simulink model "momentumBasedFlight"  (R2021b)
settings: Solver=VariableStepAuto  StartTime=0.0  StopTime=Config.simulationTime  RelTol=1e-3
InitFcn:
  | cd(fileparts(which(bdroot)));
  | initMomentumBasedFlight;
StopFcn:
  | cd(fileparts(which(bdroot)));
  | stopMomentumBasedFlight;
undefined symbols (not defined in the file or in its folder): aero_config, biasVectorConstraint_feet, Config, ConstraintMatrix_feet, DiscIntNeverNeededParam, frameNames, Frames
libraries: WBToolboxLibrary x104, momentum_flight_control_sublib x4, thrust_estimation_sublib x1, jets_control x1
(part 1 of 3)
settings Model: NumberOfSteps=50  Creator=apaolino  LastModifiedBy=icub
settings SolverCC: AlgebraicLoopSolver=TrustRegion
settings OptimizationCC: BlockReduction=off  BooleanDataType=off
settings DebuggingCC: SaveWithParameterizedLinksMsg=none  UnderspecifiedInitializationDetection=Classic  MergeDetectMultiDrivingBlocksExec=none  SignalResolutionControl=TryResolveAllWithWarning  UnconnectedInputMsg=none  UnconnectedOutputMsg=none  UnconnectedLineMsg=none
settings HardwareCC: TargetUnknown=on
settings ModelReferenceCC: EnableRefExpFcnMdlSchedulingChecks=off  PropagateSignalLabelsOutOfModel=off

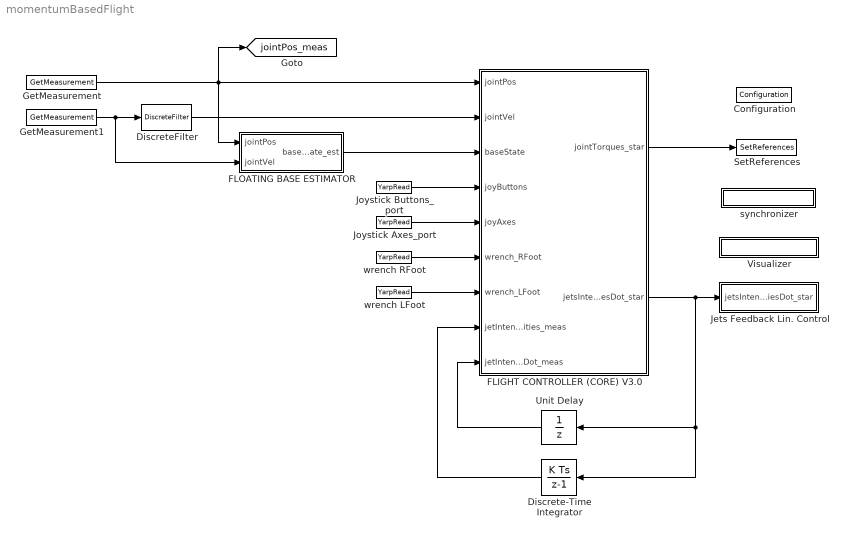
== system momentumBasedFlight ==
  Configuration : WBToolboxLibrary/Utilities/Configuration  ConfigSource=Workspace  ConfigObject='WBTConfigRobot'
      settings: SourceProductName=WholeBodyToolbox
  Discrete-Time Integrator : DiscreteIntegrator  InitialCondition=Config.initialConditions.jets_thrust  SampleTime=-1  ICPrevOutput=DiscIntNeverNeededParam  ICPrevScaledInput=DiscIntNeverNeededParam
  DiscreteFilter : WBToolboxLibrary/Utilities/DiscreteFilter  filterType=FirstOrderLowPassFilter  numCoeffs=[0]  denCoeffs=[0]  Fc=3  Ts=Config.tStep  orderMedianFilter=0  initStatus=on  y0=zeros(23,1)  u0=[0]
      settings: SourceProductName=WholeBodyToolbox
  FLIGHT CONTROLLER (CORE) V3.0 : Subsystem
  FLOATING BASE ESTIMATOR : Subsystem
  GetMeasurement : WBToolboxLibrary/States/GetMeasurement  measuredType=Joints Position
      settings: SourceProductName=WholeBodyToolbox
  GetMeasurement1 : WBToolboxLibrary/States/GetMeasurement  measuredType=Joints Velocity
      settings: SourceProductName=WholeBodyToolbox
  Jets Feedback Lin. Control : Subsystem
  Joystick Axes_port : WBToolboxLibrary/Utilities/YarpRead  portName=Ports.JOYSTICK_AXIS  signalSize=6  timeout=0.5  blocking=off  timestamp=off  autoconnect=on  errorOnConnection=off
      settings: SourceProductName=WholeBodyToolbox
  Joystick Buttons_port : WBToolboxLibrary/Utilities/YarpRead  portName=Ports.JOYSTICK_BUTTONS  signalSize=24  timeout=0.5  blocking=off  timestamp=off  autoconnect=on  errorOnConnection=off
      settings: SourceProductName=WholeBodyToolbox
  SetReferences : WBToolboxLibrary/Actuators/SetReferences  controlType=Torque  refSpeed=10*(pi/180)  refAcceleration=1000000*(pi/180)
      settings: SourceProductName=WholeBodyToolbox
  Unit Delay : UnitDelay  SampleTime=-1  HasFrameUpgradeWarning=on
  Visualizer : Subsystem
      mask Display: disp('VISUALIZER')
  synchronizer : Subsystem
      mask Display: disp('SYNCHRONIZER')
  wrench LFoot : WBToolboxLibrary/Utilities/YarpRead  portName=Ports.WRENCH_LEFT_FOOT  signalSize=6  timeout=0.5  blocking=off  timestamp=off  autoconnect=on  errorOnConnection=on
      settings: SourceProductName=WholeBodyToolbox
  wrench RFoot : WBToolboxLibrary/Utilities/YarpRead  portName=Ports.WRENCH_RIGHT_FOOT  signalSize=6  timeout=0.5  blocking=off  timestamp=off  autoconnect=on  errorOnConnection=on
      settings: SourceProductName=WholeBodyToolbox
  tag scope: jointPos_meas=global
  wires:
  GetMeasurement/1 -> FLIGHT CONTROLLER (CORE) V3.0/1(jointPos), [jointPos_meas], FLOATING BASE ESTIMATOR/1(jointPos)
  GetMeasurement1/1 -> DiscreteFilter/1, FLOATING BASE ESTIMATOR/2(jointVel)
  Joystick Buttons_port/1 -> FLIGHT CONTROLLER (CORE) V3.0/4(joyButtons)
  Joystick Axes_port/1 -> FLIGHT CONTROLLER (CORE) V3.0/5(joyAxes)
  wrench LFoot/1 -> FLIGHT CONTROLLER (CORE) V3.0/7(wrench_LFoot)
  wrench RFoot/1 -> FLIGHT CONTROLLER (CORE) V3.0/6(wrench_RFoot)
  FLIGHT CONTROLLER (CORE) V3.0/1(jointTorques_star) -> SetReferences/1
  FLIGHT CONTROLLER (CORE) V3.0/2(jetsIntensitiesDot_star) -> Jets Feedback Lin. Control/1(jetsIntensitiesDot_star), Discrete-Time Integrator/1, Unit Delay/1
  Unit Delay/1 -> FLIGHT CONTROLLER (CORE) V3.0/9(jetIntensitiesDot_meas)
  Discrete-Time Integrator/1 -> FLIGHT CONTROLLER (CORE) V3.0/8(jetIntensities_meas)
  FLOATING BASE ESTIMATOR/1(baseState_est) -> FLIGHT CONTROLLER (CORE) V3.0/3(baseState)
  DiscreteFilter/1 -> FLIGHT CONTROLLER (CORE) V3.0/2(jointVel)

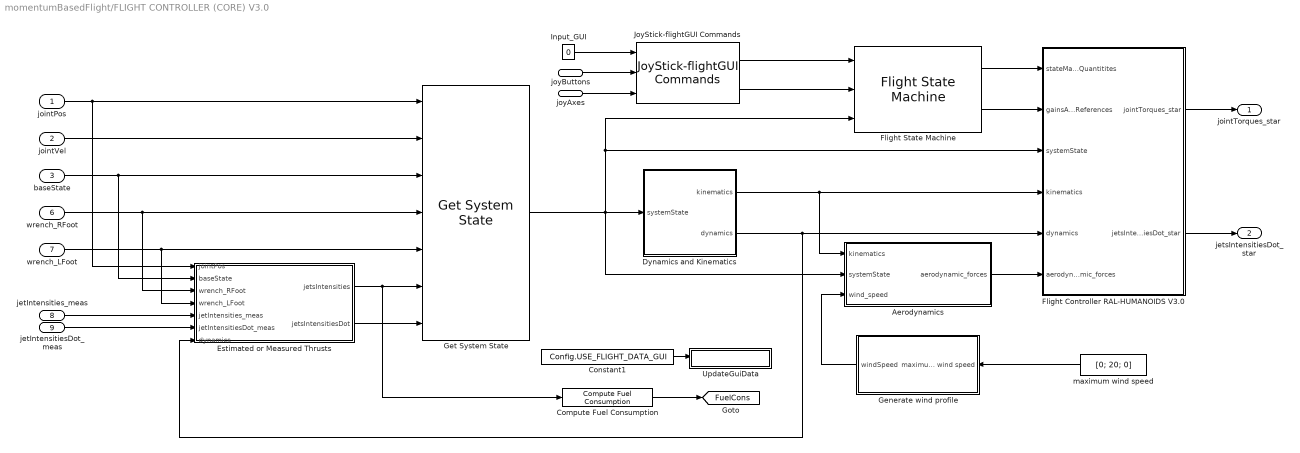
== system momentumBasedFlight/FLIGHT CONTROLLER (CORE) V3.0 ==
  jointPos : Inport
  jointVel : Inport  Port=2
  baseState : Inport  Port=3
  joyButtons : Inport  Port=4
  joyAxes : Inport  Port=5
  wrench_RFoot : Inport  Port=6
  wrench_LFoot : Inport  Port=7
  jetIntensities_meas : Inport  Port=8
  jetIntensitiesDot_meas : Inport  Port=9
  Aerodynamics : Subsystem
  Compute Fuel Consumption : momentum_flight_control_sublib/Compute Fuel Consumption  Parameter1=Config
      settings: SourceProductName=iRonCub Library
  Constant1 : Constant  Value=Config.USE_FLIGHT_DATA_GUI
  Dynamics and Kinematics : Subsystem  AncestorBlock=momentum_flight_control_sublib/Dynamics and Kinematics  mask{Parameter1=Config, Parameter2=Frames}
      mask prompts: Parameter1 "Specify the parameters struct"; Parameter2 "Specify the frame names struct"
      mask DialogControl DescGroupVar Prompt: Dynamics and Kinematics
      mask DialogControl DescTextVar Prompt: Computes the dynamics and kinematics quantities that are required by the iRonCub flight controller.
  Estimated or Measured Thrusts : Subsystem
  Flight Controller RAL-HUMANOIDS V3.0 : Subsystem  mask{Parameter1=Config}
      mask prompts: Parameter1 "Specify the parameters struct"
      mask DialogControl DescGroupVar Prompt: Flight Controller RAL-HUMANOIDS
      mask DialogControl DescTextVar Prompt: This block implements the momentum-based flight controller decribed in RAL 2018 and HUMANOIDS 2018 papers.
      mask DialogControl Control3 Prompt: References:
      mask DialogControl Control5 Prompt: RAL 2018 paper
      mask DialogControl Control5 Callback: web https://ieeexplore.ieee.org/document/7997895
      mask DialogControl Control6 Prompt: HUMANOIDS 2018 paper
      mask DialogControl Control6 Callback: web https://ieeexplore.ieee.org/document/8624985
  Flight State Machine : momentum_flight_control_sublib/Flight State Machine  Parameter1=Config  Parameter2=Frames
      settings: SourceProductName=iRonCub Library
  Generate wind profile : Subsystem
  Get System State : momentum_flight_control_sublib/Get System State  Parameter1=Frames
      settings: SourceProductName=iRonCub Library
  Input_GUI : Constant  Value=0
  JoyStick-flightGUI Commands : momentum_flight_control_sublib/JoyStick-flightGUI Commands  Parameter1=Config
      link override Input_GUI: Value=0
      settings: SourceProductName=iRonCub Library
  UpdateGuiData : Subsystem
      mask Display: disp('Update Data GUI')
  maximum wind speed : Constant  Value=[0; 20; 0]
  jointTorques_star : Outport  VectorParamsAs1DForOutWhenUnconnected=off
  jetsIntensitiesDot_star : Outport  Port=2  VectorParamsAs1DForOutWhenUnconnected=off
  tag scope: FuelCons=global
  wires:
  wrench_LFoot/1 -> Get System State/5, Estimated or Measured Thrusts/4(wrench_LFoot)
  Flight Controller RAL-HUMANOIDS V3.0/2(jetsIntensitiesDot_star) -> jetsIntensitiesDot_star/1
  Flight Controller RAL-HUMANOIDS V3.0/1(jointTorques_star) -> jointTorques_star/1
  Get System State/1 -> Dynamics and Kinematics/1(systemState), Aerodynamics/2(systemState), Flight Controller RAL-HUMANOIDS V3.0/3(systemState), Flight State Machine/3
  jointVel/1 -> Get System State/2
  jointPos/1 -> Get System State/1, Estimated or Measured Thrusts/1(jointPos)
  wrench_RFoot/1 -> Get System State/4, Estimated or Measured Thrusts/3(wrench_RFoot)
  baseState/1 -> Get System State/3, Estimated or Measured Thrusts/2(baseState)
  Compute Fuel Consumption/1 -> [FuelCons]
  JoyStick-flightGUI Commands/1 -> Flight State Machine/1
  JoyStick-flightGUI Commands/2 -> Flight State Machine/2
  Flight State Machine/1 -> Flight Controller RAL-HUMANOIDS V3.0/1(stateMachineQuantitites)
  Flight State Machine/2 -> Flight Controller RAL-HUMANOIDS V3.0/2(gainsAndReferences)
  joyAxes/1 -> JoyStick-flightGUI Commands/3
  joyButtons/1 -> JoyStick-flightGUI Commands/2
  Input_GUI/1 -> JoyStick-flightGUI Commands/1
  Constant1/1 -> UpdateGuiData/Enable
  jetIntensities_meas/1 -> Estimated or Measured Thrusts/5(jetIntensities_meas)
  jetIntensitiesDot_meas/1 -> Estimated or Measured Thrusts/6(jetIntensitiesDot_meas)
  Estimated or Measured Thrusts/1(jetsIntensities) -> Compute Fuel Consumption/1, Get System State/6
  Estimated or Measured Thrusts/2(jetsIntensitiesDot) -> Get System State/7
  Generate wind profile/1(windSpeed) -> Aerodynamics/3(wind_speed)
  maximum wind speed/1 -> Generate wind profile/1(maximum wind speed)
  Dynamics and Kinematics/2(dynamics) -> Estimated or Measured Thrusts/7(dynamics), Flight Controller RAL-HUMANOIDS V3.0/5(dynamics)
  Dynamics and Kinematics/1(kinematics) -> Flight Controller RAL-HUMANOIDS V3.0/4(kinematics), Aerodynamics/1(kinematics)
  Aerodynamics/1(aerodynamic_forces) -> Flight Controller RAL-HUMANOIDS V3.0/6(aerodynamic_forces)

== system momentumBasedFlight/FLOATING BASE ESTIMATOR ==
  jointPos : Inport
  jointVel : Inport  Port=2
  Compute State Velocity : Subsystem
  Compute base to fixed link transform : Subsystem
  Constant : Constant  Value=[1, 1]
  IMU_meas : WBToolboxLibrary/Utilities/YarpRead  portName=Ports.IMU  signalSize=Ports.IMU_PORT_SIZE  timeout=0.5  blocking=off  timestamp=off  autoconnect=on  errorOnConnection=off
      settings: SourceProductName=WholeBodyToolbox
  Terminator : Terminator
  baseState_feetFixed : MATLAB Function  TreatAsAtomicUnit=on
  baseState_est : Outport
  wires:
  IMU_meas/1 -> Compute base to fixed link transform/2(IMU_meas)
  jointPos/1 -> Compute State Velocity/1(jointPos), Compute base to fixed link transform/1(jointPos)
  jointVel/1 -> Compute State Velocity/2(jointVel)
  Constant/1 -> Compute State Velocity/4("feetContactStatus ")
  Compute base to fixed link transform/1(fixed_l_sole_H_b) -> baseState_feetFixed/2(w_H_b_yoga), Compute State Velocity/3(w_H_b)
  Compute base to fixed link transform/2(fixed_r_sole_H_b) -> Terminator/1
  Compute State Velocity/1(nu) -> baseState_feetFixed/1(nu)
  baseState_feetFixed/1(outBaseState) -> baseState_est/1

== system momentumBasedFlight/Jets Feedback Lin. Control ==
  jetsIntensitiesDot_star : Inport
  Bus Creator : BusCreator  Inputs=2
  Feedback Linearization Jets Control : jets_control/Feedback linearization 4-jets control  Conf=Config
      settings: SourceProductName=iRonCub Library
  Logical Operator : Logic  Operator=NOT  AllPortsSameDT=off  OutDataTypeStr=boolean
  "ON_GAZEBO " : Constant  Value=Config.USE_JET_DYNAMICS
  SET THROTTLE : Subsystem  Commented=on
  SET_THRUST_DERIVATIVE : Subsystem  Commented=on
  tag scope: throttle=global
  wires:
  jetsIntensitiesDot_star/1 -> Feedback Linearization Jets Control/2, SET_THRUST_DERIVATIVE/1(jetsIntensitiesDot_star)
  Feedback Linearization Jets Control/1 -> [throttle], SET THROTTLE/1(throttle)
  Bus Creator/1 -> Feedback Linearization Jets Control/1
  [jetsIntensities] -> Bus Creator/1  "jetIntensitiesFiltered"
  [jetIntensitiesDot] -> Bus Creator/2  "jetDerivativesEst"
  "ON_GAZEBO "/1 -> SET THROTTLE/Enable, Logical Operator/1
  Logical Operator/1 -> SET_THRUST_DERIVATIVE/Enable

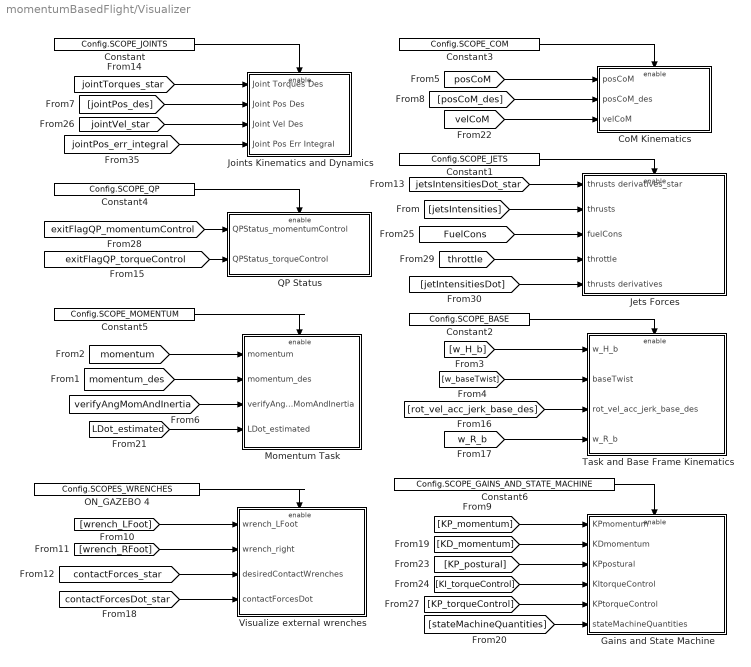
== system momentumBasedFlight/Visualizer ==
  CoM Kinematics : Subsystem
  Constant : Constant  Value=Config.SCOPE_JOINTS
  Constant1 : Constant  Value=Config.SCOPE_JETS
  Constant2 : Constant  Value=Config.SCOPE_BASE
  Constant3 : Constant  Value=Config.SCOPE_COM
  Constant4 : Constant  Value=Config.SCOPE_QP
  Constant5 : Constant  Value=Config.SCOPE_MOMENTUM
  Constant6 : Constant  Value=Config.SCOPE_GAINS_AND_STATE_MACHINE
  Gains and State Machine : Subsystem
  Jets Forces : Subsystem
  Joints Kinematics and Dynamics : Subsystem
  Momentum Task : Subsystem
  ON_GAZEBO 4 : Constant  Value=Config.SCOPES_WRENCHES
  QP Status : Subsystem
  Task and Base Frame Kinematics : Subsystem
  "Visualize external wrenches  " : Subsystem
  wires:
  [jointTorques_star] -> Joints Kinematics and Dynamics/1(Joint Torques Des)
  [jointPos_des] -> Joints Kinematics and Dynamics/2(Joint Pos Des)
  [w_H_b] -> Task and Base Frame Kinematics/1(w_H_b)
  [jointVel_star] -> Joints Kinematics and Dynamics/3(Joint Vel Des)
  Constant/1 -> Joints Kinematics and Dynamics/Enable
  [jetsIntensitiesDot_star] -> Jets Forces/1(thrusts derivatives_star)
  Constant1/1 -> Jets Forces/Enable
  [w_baseTwist] -> Task and Base Frame Kinematics/2(baseTwist)
  Constant2/1 -> Task and Base Frame Kinematics/Enable
  [momentum] -> Momentum Task/1(momentum)
  [posCoM] -> CoM Kinematics/1(posCoM)
  [posCoM_des] -> CoM Kinematics/2(posCoM_des)
  Constant3/1 -> CoM Kinematics/Enable
  [exitFlagQP_momentumControl] -> QP Status/1(QPStatus_momentumControl)
  Constant4/1 -> QP Status/Enable
  Constant5/1 -> Momentum Task/Enable
  [rot_vel_acc_jerk_base_des] -> Task and Base Frame Kinematics/3(rot_vel_acc_jerk_base_des)
  [w_R_b] -> Task and Base Frame Kinematics/4(w_R_b)
  [momentum_des] -> Momentum Task/2(momentum_des)
  [jetsIntensities] -> Jets Forces/2(thrusts)
  [verifyAngMomAndInertia] -> Momentum Task/3(verifyAngMomAndInertia)
  [wrench_LFoot] -> "Visualize external wrenches  "/1(wrench_LFoot)
  [wrench_RFoot] -> "Visualize external wrenches  "/2(wrench_right)
  ON_GAZEBO 4/1 -> "Visualize external wrenches  "/Enable
  [contactForces_star] -> "Visualize external wrenches  "/3(desiredContactWrenches)
  [exitFlagQP_torqueControl] -> QP Status/2(QPStatus_torqueControl)
  [contactForcesDot_star] -> "Visualize external wrenches  "/4(contactForcesDot)
  [LDot_estimated] -> Momentum Task/4(LDot_estimated)
  Constant6/1 -> Gains and State Machine/Enable
  [KP_momentum] -> Gains and State Machine/1(KPmomentum)
  [stateMachineQuantities] -> Gains and State Machine/6(stateMachineQuantities)
  [KD_momentum] -> Gains and State Machine/2(KDmomentum)
  [KP_postural] -> Gains and State Machine/3(KPpostural)
  [KP_torqueControl] -> Gains and State Machine/5(KPtorqueControl)
  [KI_torqueControl] -> Gains and State Machine/4(KItorqueControl)
  [jointPos_err_integral] -> Joints Kinematics and Dynamics/4(Joint Pos Err Integral)
  [velCoM] -> CoM Kinematics/3(velCoM)
  [FuelCons] -> Jets Forces/3(fuelCons)
  [throttle] -> Jets Forces/4(throttle)
  [jetIntensitiesDot] -> Jets Forces/5(thrusts derivatives)

== system momentumBasedFlight/synchronizer ==
  GAZEBO_SYNCHRONIZER : Subsystem
  Logical Operator : Logic  Operator=NOT  AllPortsSameDT=off  OutDataTypeStr=boolean
  "ON_GAZEBO " : Constant  Value=Config.ON_GAZEBO
  REAL_TIME_SYNC : Subsystem
  wires:
  Logical Operator/1 -> REAL_TIME_SYNC/Enable
  "ON_GAZEBO "/1 -> GAZEBO_SYNCHRONIZER/Enable, Logical Operator/1

== system momentumBasedFlight/FLIGHT CONTROLLER (CORE) V3.0/Aerodynamics ==
  kinematics : Inport
  systemState : Inport  Port=2
  wind_speed : Inport  Port=3
  Bus Selector : BusSelector  OutputSignals=w_baseTwist,jointVel
  Bus Selector1 : BusSelector  OutputSignals=J_aeroForce,matrixOfLinkCoMTransform
  Terminator : Terminator
  aeroDyn : MATLABSystem  System=aeroDyn  aero_config=aero_config_with_frames  SimulateUsing=Interpreted execution
      mask Type: aeroDyn
      mask Display:
      | disp('aeroDyn');
      | port_label('input',1,'base_velocity');
      | port_label('input',2,'joints_velocity');
      | port_label('input',3,'wind_speed');
      | port_label('input',4,'J_aeroForce');
      | port_label('input',5,'matrixOfAeroTransform');
      | port_label('output',1,'aerodynamic_forces');
      | port_label('output',2,'generalized_aerodynamic_wrench');
  aerodynamic_forces : Outport
  wires:
  systemState/1 -> Bus Selector/1
  Bus Selector/1 -> aeroDyn/1  "<w_baseTwist>"
  aeroDyn/1 -> aerodynamic_forces/1  "aerodynamic_forces"
  aeroDyn/2 -> Terminator/1
  kinematics/1 -> Bus Selector1/1
  Bus Selector1/1 -> aeroDyn/4  "<J_aeroForce>"
  Bus Selector1/2 -> aeroDyn/5  "<matrixOfLinkCoMTransform>"
  Bus Selector/2 -> aeroDyn/2  "<jointVel>"
  wind_speed/1 -> aeroDyn/3

== system momentumBasedFlight/FLIGHT CONTROLLER (CORE) V3.0/Dynamics and Kinematics ==
  systemState : Inport
  Bus Creator1 : BusCreator  Inputs=5
  Bus Creator2 : BusCreator  Inputs=15
  Bus Selector : BusSelector  OutputSignals=w_H_b,jointPos,w_baseTwist,jointVel
  Dynamic Quantities : Subsystem
  Kinematic Quantities : Subsystem
  kinematics : Outport  VectorParamsAs1DForOutWhenUnconnected=off
  dynamics : Outport  Port=2  VectorParamsAs1DForOutWhenUnconnected=off
  wires:
  Dynamic Quantities/5(w_I_c) -> Bus Creator1/5  "w_I_c"
  Kinematic Quantities/12(posCoM) -> Dynamic Quantities/1(posCoM), Bus Creator2/12  "posCoM"
  Kinematic Quantities/11(matrixOfJetsArms) -> Bus Creator2/11  "matrixOfJetsArms"
  Kinematic Quantities/10(matrixOfJetsAxes) -> Bus Creator2/10  "matrixOfJetAxes"
  Kinematic Quantities/9(w_H_RFoot) -> Bus Creator2/9  "w_H_RFoot"
  Kinematic Quantities/8(w_H_LFoot) -> Bus Creator2/8  "w_H_LFoot"
  Kinematic Quantities/7(JDot_RFoot_nu) -> Bus Creator2/7  "JDot_RFoot_nu"
  Kinematic Quantities/6(JDot_LFoot_nu) -> Bus Creator2/6  "JDot_LFoot_nu"
  Kinematic Quantities/5(J_RFoot) -> Bus Creator2/5  "J_RFoot"
  Kinematic Quantities/4(J_LFoot) -> Bus Creator2/4  "J_LFoot"
  Kinematic Quantities/3(w_R_b) -> Bus Creator2/3  "w_R_b"
  Kinematic Quantities/2(J_CoM) -> Bus Creator2/2  "J_CoM"
  Kinematic Quantities/1(J_jets) -> Bus Creator2/1  "J_jets"
  Bus Creator2/1 -> kinematics/1
  Bus Creator1/1 -> dynamics/1
  Dynamic Quantities/1(M) -> Bus Creator1/1  "M"
  Dynamic Quantities/2("h ") -> Bus Creator1/2  "h"
  Dynamic Quantities/3(L) -> Bus Creator1/3  "L"
  Dynamic Quantities/4(CMM) -> Bus Creator1/4  "CMM"
  Bus Selector/4 -> Kinematic Quantities/4(jointVel), Dynamic Quantities/5(jointVel)  "<jointVel>"
  Bus Selector/3 -> Kinematic Quantities/3(w_baseTwist), Dynamic Quantities/4(w_baseTwist)  "<w_baseTwist>"
  Bus Selector/2 -> Kinematic Quantities/2(jointPos), Dynamic Quantities/3(jointPos)  "<jointPos>"
  Bus Selector/1 -> Kinematic Quantities/1(w_H_b), Dynamic Quantities/2(w_H_b)  "<w_H_b>"
  systemState/1 -> Bus Selector/1
  Kinematic Quantities/13(matrixOfAeroArms) -> Bus Creator2/13
  Kinematic Quantities/14(J_aeroForces) -> Bus Creator2/14  "J_aeroForce"
  Kinematic Quantities/15(matrixOfAeroTransform) -> Bus Creator2/15

== system momentumBasedFlight/FLIGHT CONTROLLER (CORE) V3.0/Estimated or Measured Thrusts ==
  jointPos : Inport
  baseState : Inport  Port=2
  wrench_RFoot : Inport  Port=3
  wrench_LFoot : Inport  Port=4
  jetIntensities_meas : Inport  Port=5
  jetIntensitiesDot_meas : Inport  Port=6
  dynamics : Inport  Port=7
  " Thrust Estimator" : Subsystem
  "ON_GAZEBO " : Constant  Value=Config.USE_JET_DYNAMICS
  ON_GAZEBO 1 : Constant  Value=Config.USE_THRUST_ESTIMATOR
  Selector1 : Selector  InputPortWidth=18  IndexOptions=Index vector (dialog)  Indices=[1:6]  OutputSizes=1
  Switch : Switch  Criteria=u2 > Threshold
  Switch1 : Switch  Criteria=u2 > Threshold
  fromPosRPYtoTransfMatrix : MATLAB Function  TreatAsAtomicUnit=on
  jetsIntensities : Outport
  jetsIntensitiesDot : Outport  Port=2
  wires:
  Switch/1 -> jetsIntensities/1  "jetsIntensities"
  jetIntensitiesDot_meas/1 -> Switch1/3
  " Thrust Estimator"/1(jetIntensities_Estimated) -> Switch/1
  jetIntensities_meas/1 -> Switch/3
  " Thrust Estimator"/2(jetIntensitiesDot_Estimated) -> Switch1/1
  wrench_RFoot/1 -> " Thrust Estimator"/5(wrench_RFoot)
  ON_GAZEBO 1/1 -> Switch/2, Switch1/2
  jointPos/1 -> " Thrust Estimator"/2(jointPos)
  Switch1/1 -> jetsIntensitiesDot/1  "jetsIntensitiesDot"
  dynamics/1 -> " Thrust Estimator"/3(dynamics)
  [throttle] -> " Thrust Estimator"/6(throttle)
  "ON_GAZEBO "/1 -> " Thrust Estimator"/Enable
  wrench_LFoot/1 -> " Thrust Estimator"/4(wrench_LFoot)
  baseState/1 -> Selector1/1
  fromPosRPYtoTransfMatrix/1(w_H_b) -> " Thrust Estimator"/1(w_H_b)
  Selector1/1 -> fromPosRPYtoTransfMatrix/1(pos_rpy)

== system momentumBasedFlight/FLIGHT CONTROLLER (CORE) V3.0/Flight Controller RAL-HUMANOIDS V3.0 ==
  stateMachineQuantitites : Inport
  gainsAndReferences : Inport  Port=2
  systemState : Inport  Port=3
  kinematics : Inport  Port=4
  dynamics : Inport  Port=5
  aerodynamic_forces : Inport  Port=6
  Discrete-Time Integrator : DiscreteIntegrator  Commented=on  InitialConditionSource=external  SampleTime=Config.tStep  ICPrevOutput=DiscIntNeverNeededParam  ICPrevScaledInput=DiscIntNeverNeededParam
  GetMeasurement : WBToolboxLibrary/States/GetMeasurement  Commented=on  measuredType=Joints Position
      settings: SourceProductName=WholeBodyToolbox
  Joint Torque Control for Flying : Subsystem
  Momentum Control for Flying : Subsystem
  SetReferences : WBToolboxLibrary/Actuators/SetReferences  Commented=on  controlType=Position Direct  refSpeed=10*(pi/180)  refAcceleration=1000000*(pi/180)
      settings: SourceProductName=WholeBodyToolbox
  deadZone : Subsystem  Commented=on
  "holder " : WBToolboxLibrary/Utilities/holder   Commented=on
      settings: SourceProductName=WholeBodyToolbox
  jointTorques_star : Outport  VectorParamsAs1DForOutWhenUnconnected=off
  jetsIntensitiesDot_star : Outport  Port=2  VectorParamsAs1DForOutWhenUnconnected=off
  tag scope: jointTorques_star=global
  wires:
  Momentum Control for Flying/3(jetsIntensitiesDot_star) -> jetsIntensitiesDot_star/1
  Joint Torque Control for Flying/1(jointTorques_star) -> [jointTorques_star], jointTorques_star/1
  Momentum Control for Flying/2(contactForces_star) -> Joint Torque Control for Flying/2(contactForces_star)
  dynamics/1 -> Momentum Control for Flying/5(dynamics), Joint Torque Control for Flying/7(dynamics)
  kinematics/1 -> Momentum Control for Flying/4(kinematics), Joint Torque Control for Flying/6(kinematics)
  systemState/1 -> Momentum Control for Flying/3(systemState), Joint Torque Control for Flying/5(systemState)
  gainsAndReferences/1 -> Joint Torque Control for Flying/4(gainsAndReferences), Momentum Control for Flying/2(gainsAndReferences)
  stateMachineQuantitites/1 -> Joint Torque Control for Flying/3(stateMachineQuantitites), Momentum Control for Flying/1(stateMachineQuantitites)
  aerodynamic_forces/1 -> Joint Torque Control for Flying/8(aerodynamic_forces), Momentum Control for Flying/6(aerodynamic_forces)
  "holder "/1 -> Discrete-Time Integrator/2
  Discrete-Time Integrator/1 -> SetReferences/1
  GetMeasurement/1 -> "holder "/1
  deadZone/1(u_cut) -> Discrete-Time Integrator/1
  Momentum Control for Flying/1(jointVel_star) -> Joint Torque Control for Flying/1(jointVel_star), deadZone/1(u)

== system momentumBasedFlight/FLIGHT CONTROLLER (CORE) V3.0/Generate wind profile ==
  maximum wind speed : Inport
  Clock : Clock
  Constant1 : Constant  Value=aero_config.USE_WIND_SPEED
  MATLAB Function : MATLAB Function  TreatAsAtomicUnit=on
  Switch1 : Switch  Criteria=u2 ~= 0
  wind speed : Scope
  zero_wind_speed : Constant  Value=zeros(3,1)
  windSpeed : Outport
  tag scope: windSpeed=global
  wires:
  Clock/1 -> MATLAB Function/2(time)
  zero_wind_speed/1 -> Switch1/3
  maximum wind speed/1 -> MATLAB Function/1(maxWindSpeed)
  MATLAB Function/1(windSpeed) -> wind speed/1, [windSpeed], Switch1/1
  Constant1/1 -> Switch1/2
  Switch1/1 -> windSpeed/1

== system momentumBasedFlight/FLIGHT CONTROLLER (CORE) V3.0/UpdateGuiData ==
  Enable : EnablePort
  Clock : Clock
  Update Data for the GUI : MATLAB Function  TreatAsAtomicUnit=on
  wires:
  Clock/1 -> Update Data for the GUI/1(time)

== system momentumBasedFlight/FLOATING BASE ESTIMATOR/Compute State Velocity ==
  jointPos : Inport
  jointVel : Inport  Port=2
  w_H_b : Inport  Port=3
  "feetContactStatus " : Inport  Port=4
  Compute Base Velocity : MATLAB Function  TreatAsAtomicUnit=on
  Feet Jacobians : Subsystem
  Mux : Mux  Inputs=2
  nu : Outport  VectorParamsAs1DForOutWhenUnconnected=off
  wires:
  jointVel/1 -> Mux/2, Compute Base Velocity/4(jointVel)
  Mux/1 -> nu/1
  "feetContactStatus "/1 -> Compute Base Velocity/3(feetContactStatus)
  Compute Base Velocity/1(nu_b) -> Mux/1
  jointPos/1 -> Feet Jacobians/1(jointPos)
  w_H_b/1 -> Feet Jacobians/2(w_H_b)
  Feet Jacobians/1(J_l_sole) -> Compute Base Velocity/1(J_l_sole)
  Feet Jacobians/2(J_r_sole) -> Compute Base Velocity/2(J_r_sole)

== system momentumBasedFlight/FLOATING BASE ESTIMATOR/Compute base to fixed link transform ==
  jointPos : Inport
  IMU_meas : Inport  Port=2
  Constant7 : Constant  Value=eye(4)
  "LFoot to base link transform " : Subsystem
  RFoot to base link transform : Subsystem
  Relative transform l_sole_H_base : WBToolboxLibrary/Model/Kinematics/ForwardKinematics  frameName=Frames.LFOOT_FRAME
      settings: SourceProductName=WholeBodyToolbox
  Relative transform r_sole_H_base : WBToolboxLibrary/Model/Kinematics/ForwardKinematics  frameName=Frames.RFOOT_FRAME
      settings: SourceProductName=WholeBodyToolbox
  fixed_l_sole_H_b : Outport  VectorParamsAs1DForOutWhenUnconnected=off
  fixed_r_sole_H_b : Outport  Port=2  VectorParamsAs1DForOutWhenUnconnected=off
  wires:
  Constant7/1 -> RFoot to base link transform/4(w_H_base_fixed), "LFoot to base link transform "/4(w_H_base_fixed), Relative transform r_sole_H_base/1, Relative transform l_sole_H_base/1
  RFoot to base link transform/1(link_H_b) -> fixed_r_sole_H_b/1
  "LFoot to base link transform "/1(link_H_b) -> fixed_l_sole_H_b/1
  Relative transform l_sole_H_base/1 -> "LFoot to base link transform "/3(w_H_link)
  Relative transform r_sole_H_base/1 -> RFoot to base link transform/3(w_H_link)
  jointPos/1 -> RFoot to base link transform/1(jointPos), "LFoot to base link transform "/1(jointPos), Relative transform r_sole_H_base/2, Relative transform l_sole_H_base/2
  IMU_meas/1 -> RFoot to base link transform/2(inertial), "LFoot to base link transform "/2(inertial)

== system momentumBasedFlight/Jets Feedback Lin. Control/SET THROTTLE ==
  throttle : Inport
  Enable : EnablePort
  Set Throttle : WBToolboxLibrary/Utilities/YarpWrite  portName=Ports.THROTTLE  autoconnect=on  errorOnConnection=on
      settings: SourceProductName=WholeBodyToolbox
  wires:
  throttle/1 -> Set Throttle/1

== system momentumBasedFlight/Jets Feedback Lin. Control/SET_THRUST_DERIVATIVE ==
  jetsIntensitiesDot_star : Inport
  Enable : EnablePort
  Set Thrust Derivative : WBToolboxLibrary/Utilities/YarpWrite  portName=Ports.THRUST_RATIO  autoconnect=on  errorOnConnection=on
      settings: SourceProductName=WholeBodyToolbox
  wires:
  jetsIntensitiesDot_star/1 -> Set Thrust Derivative/1

== system momentumBasedFlight/Visualizer/CoM Kinematics ==
  posCoM : Inport
  posCoM_des : Inport  Port=2
  velCoM : Inport  Port=3
  Enable : EnablePort
  CoM position : Scope  NumInputPorts=3
  CoM position desired : Scope  NumInputPorts=3
  CoM position error : Scope  NumInputPorts=3
  CoM velocity : Scope  NumInputPorts=3
  Demux{1..3,8} (4 alike) : Demux  Outputs=3
  Mux : Mux  Inputs=2
  Mux1 : Mux  Inputs=2
  Mux2 : Mux  Inputs=2
  Sum : Sum  Inputs=+-|
  Task CoM combined : Scope  NumInputPorts=3
  wires:
  posCoM/1 -> Sum/1, Demux8/1
  posCoM_des/1 -> Sum/2, Demux1/1
  Sum/1 -> Demux2/1
  Demux2/3 -> CoM position error/3  "CoM_z"
  Demux2/2 -> CoM position error/2  "CoM_y"
  Demux2/1 -> CoM position error/1  "CoM_x"
  Demux8/2 -> CoM position/2, Mux1/1  "yCoM"
  Demux1/2 -> Mux1/2, CoM position desired/2  "yCoM des"
  Mux2/1 -> Task CoM combined/3
  Demux8/1 -> CoM position/1, Mux/1  "xCoM"
  Demux8/3 -> CoM position/3, Mux2/1  "zCoM"
  Mux1/1 -> Task CoM combined/2
  Demux1/1 -> CoM position desired/1, Mux/2  "xCoM des"
  Demux1/3 -> CoM position desired/3, Mux2/2  "zCoM des"
  Mux/1 -> Task CoM combined/1
  velCoM/1 -> Demux3/1
  Demux3/1 -> CoM velocity/1  "CoM_x"
  Demux3/2 -> CoM velocity/2  "CoM_y"
  Demux3/3 -> CoM velocity/3  "CoM_z"

== system momentumBasedFlight/Visualizer/Gains and State Machine ==
  KPmomentum : Inport
  KDmomentum : Inport  Port=2
  KPpostural : Inport  Port=3
  KItorqueControl : Inport  Port=4
  KPtorqueControl : Inport  Port=5
  stateMachineQuantities : Inport  Port=6
  Enable : EnablePort
  Bus Selector1 : BusSelector  OutputSignals=decreaseMaxFootVerticalForce,increaseMinFootVerticalForce,feetContactIsActive,robotIsLanded,oneFootIsInContact
  Feet Are in Contact : Scope
  KD_momentum : Scope
  KI_torqueControl : Scope
  KP_momentum : Scope
  KP_postural : Scope
  KP_torqueControl : Scope
  One Foot Is In Contact : Scope
  Robot Is Landed : Scope
  Start Flying Procedure : Scope
  Start Landing Procedure : Scope
  wires:
  stateMachineQuantities/1 -> Bus Selector1/1
  Bus Selector1/1 -> Start Flying Procedure/1  "<decreaseMaxFootVerticalForce>"
  Bus Selector1/2 -> Start Landing Procedure/1  "<increaseMinFootVerticalForce>"
  Bus Selector1/3 -> Feet Are in Contact/1  "<feetContactIsActive>"
  KPmomentum/1 -> KP_momentum/1
  KDmomentum/1 -> KD_momentum/1
  KPpostural/1 -> KP_postural/1
  KItorqueControl/1 -> KI_torqueControl/1
  KPtorqueControl/1 -> KP_torqueControl/1
  Bus Selector1/4 -> Robot Is Landed/1  "<robotIsLanded>"
  Bus Selector1/5 -> One Foot Is In Contact/1  "<oneFootIsInContact>"

== system momentumBasedFlight/Visualizer/Jets Forces ==
  thrusts derivatives_star : Inport
  thrusts : Inport  Port=2
  fuelCons : Inport  Port=3
  throttle : Inport  Port=4
  thrusts derivatives : Inport  Port=5
  Enable : EnablePort
  Fuel Consumption : Scope
  throttle input : Scope
  thrust : Scope
  thrust derivatives : Scope
  thrust derivatives_star : Scope
  wires:
  thrusts derivatives_star/1 -> thrust derivatives_star/1
  thrusts/1 -> thrust/1
  fuelCons/1 -> Fuel Consumption/1
  throttle/1 -> throttle input/1
  thrusts derivatives/1 -> thrust derivatives/1

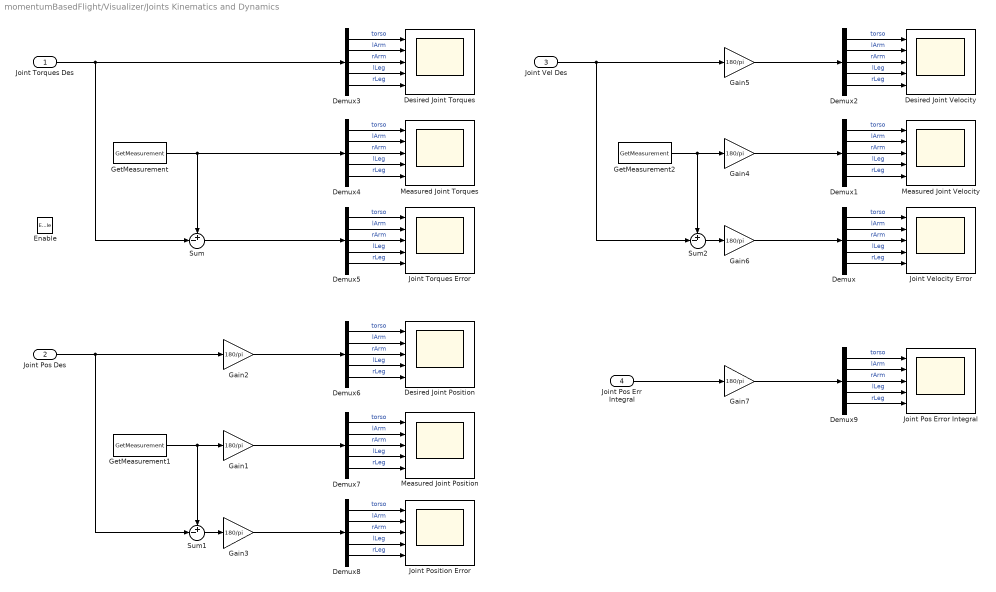
== system momentumBasedFlight/Visualizer/Joints Kinematics and Dynamics ==
  Joint Torques Des : Inport
  Joint Pos Des : Inport  Port=2
  Joint Vel Des : Inport  Port=3
  Joint Pos Err Integral : Inport  Port=4
  Enable : EnablePort
  Demux{,1..9} (10 alike) : Demux  Outputs=Config.numOfJointsForEachControlboard
  Desired Joint Position : Scope  NumInputPorts=5
  Desired Joint Torques : Scope  NumInputPorts=5
  Desired Joint Velocity : Scope  NumInputPorts=5
  Gain{1..7} (7 alike) : Gain  Gain=180/pi
  GetMeasurement : WBToolboxLibrary/States/GetMeasurement  measuredType=Joints Torque
      settings: SourceProductName=WholeBodyToolbox
  GetMeasurement1 : WBToolboxLibrary/States/GetMeasurement  measuredType=Joints Position
      settings: SourceProductName=WholeBodyToolbox
  GetMeasurement2 : WBToolboxLibrary/States/GetMeasurement  measuredType=Joints Velocity
      settings: SourceProductName=WholeBodyToolbox
  Joint Pos Error Integral : Scope  NumInputPorts=5
  Joint Position Error : Scope  NumInputPorts=5
  Joint Torques Error : Scope  NumInputPorts=5
  Joint Velocity Error : Scope  NumInputPorts=5
  Measured Joint Position : Scope  NumInputPorts=5
  Measured Joint Torques : Scope  NumInputPorts=5
  Measured Joint Velocity : Scope  NumInputPorts=5
  Sum : Sum  Inputs=+-|
  Sum1 : Sum  Inputs=+-|
  Sum2 : Sum  Inputs=+-|
  wires:
  Demux5/3 -> Joint Torques Error/3  "rArm"
  Demux5/4 -> Joint Torques Error/4  "lLeg"
  Demux5/5 -> Joint Torques Error/5  "rLeg"
  Sum/1 -> Demux5/1
  Demux5/1 -> Joint Torques Error/1  "torso"
  Demux5/2 -> Joint Torques Error/2  "lArm"
  GetMeasurement/1 -> Demux4/1, Sum/1
  Demux4/3 -> Measured Joint Torques/3  "rArm"
  Demux4/2 -> Measured Joint Torques/2  "lArm"
  Demux4/5 -> Measured Joint Torques/5  "rLeg"
  Demux4/4 -> Measured Joint Torques/4  "lLeg"
  Demux4/1 -> Measured Joint Torques/1  "torso"
  Demux3/1 -> Desired Joint Torques/1  "torso"
  Demux3/5 -> Desired Joint Torques/5  "rLeg"
  Joint Torques Des/1 -> Demux3/1, Sum/2
  Demux3/3 -> Desired Joint Torques/3  "rArm"
  Demux3/2 -> Desired Joint Torques/2  "lArm"
  Demux3/4 -> Desired Joint Torques/4  "lLeg"
  Demux7/4 -> Measured Joint Position/4  "lLeg"
  Demux7/2 -> Measured Joint Position/2  "lArm"
  Joint Pos Des/1 -> Sum1/2, Gain2/1
  Demux8/2 -> Joint Position Error/2  "lArm"
  Sum1/1 -> Gain3/1
  Demux7/1 -> Measured Joint Position/1  "torso"
  Demux8/5 -> Joint Position Error/5  "rLeg"
  GetMeasurement1/1 -> Sum1/1, Gain1/1
  Demux8/4 -> Joint Position Error/4  "lLeg"
  Demux6/1 -> Desired Joint Position/1  "torso"
  Demux8/3 -> Joint Position Error/3  "rArm"
  Demux6/2 -> Desired Joint Position/2  "lArm"
  Demux6/4 -> Desired Joint Position/4  "lLeg"
  Demux7/5 -> Measured Joint Position/5  "rLeg"
  Demux6/5 -> Desired Joint Position/5  "rLeg"
  Demux8/1 -> Joint Position Error/1  "torso"
  Demux7/3 -> Measured Joint Position/3  "rArm"
  Demux6/3 -> Desired Joint Position/3  "rArm"
  Gain1/1 -> Demux7/1
  Gain2/1 -> Demux6/1
  Gain3/1 -> Demux8/1
  Joint Vel Des/1 -> Sum2/2, Gain5/1
  Demux2/3 -> Desired Joint Velocity/3  "rArm"
  Demux/3 -> Joint Velocity Error/3  "rArm"
  Demux2/1 -> Desired Joint Velocity/1  "torso"
  Demux2/5 -> Desired Joint Velocity/5  "rLeg"
  Demux2/4 -> Desired Joint Velocity/4  "lLeg"
  Demux1/5 -> Measured Joint Velocity/5  "rLeg"
  Demux1/1 -> Measured Joint Velocity/1  "torso"
  Demux/5 -> Joint Velocity Error/5  "rLeg"
  Gain4/1 -> Demux1/1
  Demux/2 -> Joint Velocity Error/2  "lArm"
  Demux/1 -> Joint Velocity Error/1  "torso"
  Demux/4 -> Joint Velocity Error/4  "lLeg"
  Sum2/1 -> Gain6/1
  Demux1/2 -> Measured Joint Velocity/2  "lArm"
  Demux1/4 -> Measured Joint Velocity/4  "lLeg"
  Demux2/2 -> Desired Joint Velocity/2  "lArm"
  Demux1/3 -> Measured Joint Velocity/3  "rArm"
  Gain6/1 -> Demux/1
  Gain5/1 -> Demux2/1
  GetMeasurement2/1 -> Sum2/1, Gain4/1
  Demux9/1 -> Joint Pos Error Integral/1  "torso"
  Demux9/5 -> Joint Pos Error Integral/5  "rLeg"
  Joint Pos Err Integral/1 -> Gain7/1
  Gain7/1 -> Demux9/1
  Demux9/3 -> Joint Pos Error Integral/3  "rArm"
  Demux9/2 -> Joint Pos Error Integral/2  "lArm"
  Demux9/4 -> Joint Pos Error Integral/4  "lLeg"

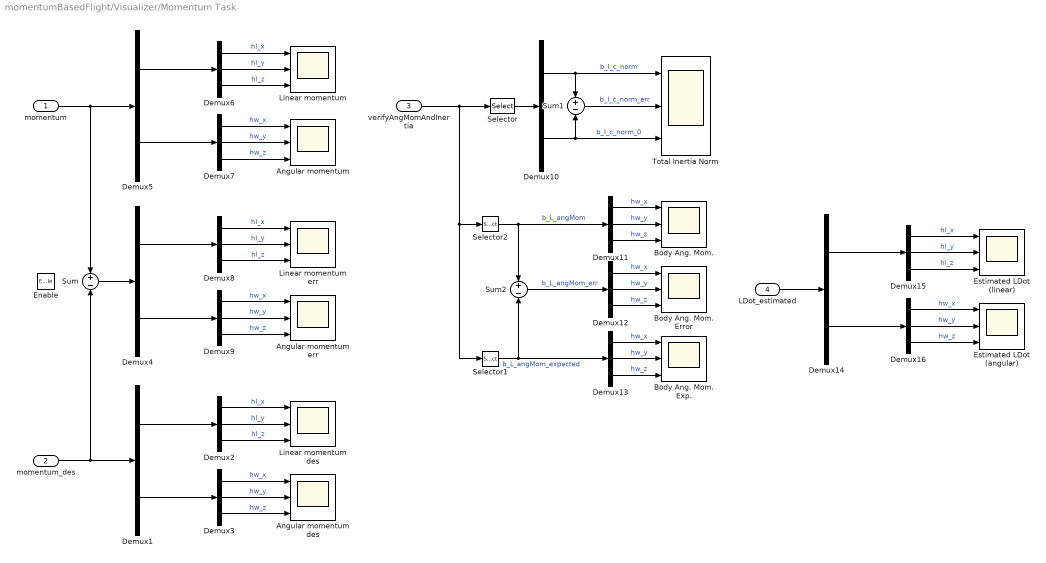
== system momentumBasedFlight/Visualizer/Momentum Task ==
  momentum : Inport
  momentum_des : Inport  Port=2
  verifyAngMomAndInertia : Inport  Port=3
  LDot_estimated : Inport  Port=4
  Enable : EnablePort
  Angular momentum : Scope  NumInputPorts=3
  Angular momentum des : Scope  NumInputPorts=3
  Angular momentum err : Scope  NumInputPorts=3
  Body Ang. Mom. : Scope  NumInputPorts=3
  Body Ang. Mom. Error : Scope  NumInputPorts=3
  Body Ang. Mom. Exp. : Scope  NumInputPorts=3
  Demux{1,4..5,10,14} (5 alike) : Demux  Outputs=2
  Demux{2..3,6..9,11..13,15..16} (11 alike) : Demux  Outputs=3
  Estimated LDot (angular) : Scope  NumInputPorts=3
  Estimated LDot (linear) : Scope  NumInputPorts=3
  Linear momentum : Scope  NumInputPorts=3
  Linear momentum des : Scope  NumInputPorts=3
  Linear momentum err : Scope  NumInputPorts=3
  Selector : Selector  NumberOfDimensions=2  InputPortWidth=3  IndexOptions=Index vector (dialog),Index vector (dialog)  Indices=[1],[1 2]  OutputSizes=1,1
  Selector1 : Selector  NumberOfDimensions=2  InputPortWidth=3  IndexOptions=Index vector (dialog),Index vector (dialog)  Indices=[2 3 4],[2]  OutputSizes=1,1
  Selector2 : Selector  NumberOfDimensions=2  InputPortWidth=3  IndexOptions=Index vector (dialog),Index vector (dialog)  Indices=[2 3 4],[1]  OutputSizes=1,1
  Sum : Sum  Inputs=+|-
  Sum1 : Sum  Inputs=+|-
  Sum2 : Sum  Inputs=+|-
  Total Inertia Norm : Scope  NumInputPorts=3
  wires:
  Demux6/1 -> Linear momentum/1  "hl_x"
  Demux6/3 -> Linear momentum/3  "hl_z"
  Demux5/2 -> Demux7/1
  Demux6/2 -> Linear momentum/2  "hl_y"
  Demux5/1 -> Demux6/1
  Demux7/1 -> Angular momentum/1  "hw_x"
  Demux7/3 -> Angular momentum/3  "hw_z"
  Demux7/2 -> Angular momentum/2  "hw_y"
  momentum/1 -> Sum/1, Demux5/1
  Demux3/2 -> Angular momentum des/2  "hw_y"
  Demux3/1 -> Angular momentum des/1  "hw_x"
  Demux2/3 -> Linear momentum des/3  "hl_z"
  Demux2/1 -> Linear momentum des/1  "hl_x"
  Demux1/2 -> Demux3/1
  Demux1/1 -> Demux2/1
  Demux3/3 -> Angular momentum des/3  "hw_z"
  Demux2/2 -> Linear momentum des/2  "hl_y"
  momentum_des/1 -> Sum/2, Demux1/1
  Demux9/2 -> Angular momentum err/2  "hw_y"
  Demux9/1 -> Angular momentum err/1  "hw_x"
  Demux8/3 -> Linear momentum err/3  "hl_z"
  Demux8/1 -> Linear momentum err/1  "hl_x"
  Demux4/2 -> Demux9/1
  Demux4/1 -> Demux8/1
  Demux9/3 -> Angular momentum err/3  "hw_z"
  Demux8/2 -> Linear momentum err/2  "hl_y"
  Sum/1 -> Demux4/1
  verifyAngMomAndInertia/1 -> Selector/1, Selector1/1, Selector2/1
  Selector/1 -> Demux10/1
  Demux10/1 -> Total Inertia Norm/1, Sum1/1  "b_I_c_norm"
  Demux10/2 -> Total Inertia Norm/3, Sum1/2  "b_I_c_norm_0"
  Sum1/1 -> Total Inertia Norm/2  "b_I_c_norm_err"
  Selector2/1 -> Demux11/1, Sum2/1  "b_L_angMom"
  Demux11/2 -> Body Ang. Mom./2  "hw_y"
  Demux11/3 -> Body Ang. Mom./3  "hw_z"
  Demux11/1 -> Body Ang. Mom./1  "hw_x"
  Demux12/2 -> Body Ang. Mom. Error/2  "hw_y"
  Sum2/1 -> Demux12/1  "b_L_angMom_err"
  Demux12/3 -> Body Ang. Mom. Error/3  "hw_z"
  Demux12/1 -> Body Ang. Mom. Error/1  "hw_x"
  Demux13/2 -> Body Ang. Mom. Exp./2  "hw_y"
  Selector1/1 -> Sum2/2, Demux13/1  "b_L_angMom_expected"
  Demux13/3 -> Body Ang. Mom. Exp./3  "hw_z"
  Demux13/1 -> Body Ang. Mom. Exp./1  "hw_x"
  LDot_estimated/1 -> Demux14/1
  Demux15/3 -> Estimated LDot (linear)/3  "hl_z"
  Demux16/2 -> Estimated LDot (angular)/2  "hw_y"
  Demux14/1 -> Demux15/1
  Demux14/2 -> Demux16/1
  Demux15/2 -> Estimated LDot (linear)/2  "hl_y"
  Demux15/1 -> Estimated LDot (linear)/1  "hl_x"
  Demux16/1 -> Estimated LDot (angular)/1  "hw_x"
  Demux16/3 -> Estimated LDot (angular)/3  "hw_z"

== system momentumBasedFlight/Visualizer/QP Status ==
  QPStatus_momentumControl : Inport
  QPStatus_torqueControl : Inport  Port=2
  Enable : EnablePort
  QP momentum : Scope
  QP torques : Scope
  wires:
  QPStatus_momentumControl/1 -> QP momentum/1
  QPStatus_torqueControl/1 -> QP torques/1

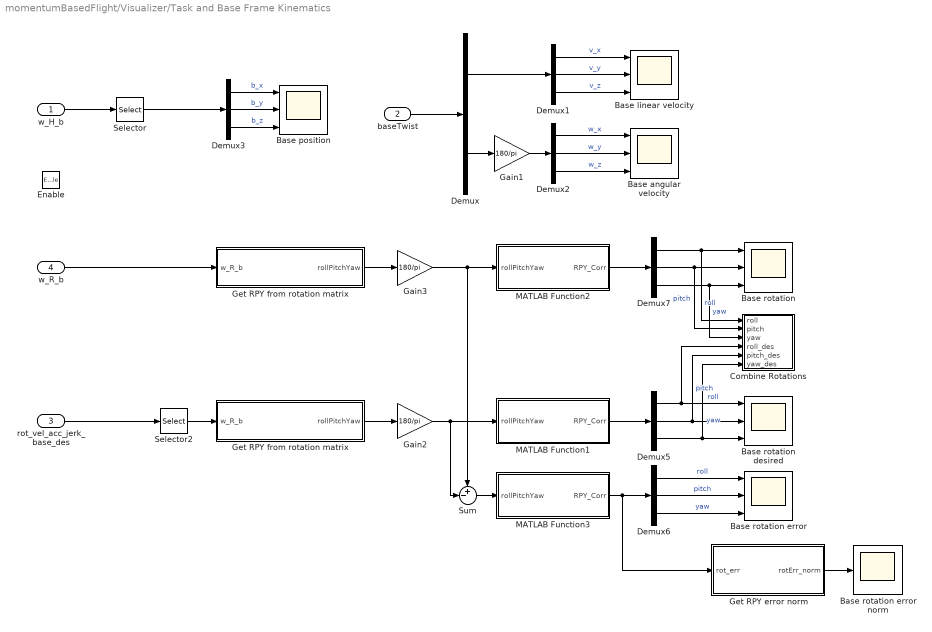
== system momentumBasedFlight/Visualizer/Task and Base Frame Kinematics ==
  w_H_b : Inport
  baseTwist : Inport  Port=2
  rot_vel_acc_jerk_base_des : Inport  Port=3
  w_R_b : Inport  Port=4
  Enable : EnablePort
  Base angular velocity : Scope  NumInputPorts=3
  Base linear velocity : Scope  NumInputPorts=3
  Base position : Scope  NumInputPorts=3
  Base rotation : Scope  NumInputPorts=3
  Base rotation desired : Scope  NumInputPorts=3
  Base rotation error : Scope  NumInputPorts=3
  Base rotation error norm : Scope
  Combine Rotations : Subsystem
  Demux : Demux  Outputs=2
  Demux{1..3,5..7} (6 alike) : Demux  Outputs=3
  Gain1 : Gain  Gain=180/pi
  Gain2 : Gain  Gain=180/pi
  Gain3 : Gain  Gain=180/pi
  Get RPY error norm : MATLAB Function  TreatAsAtomicUnit=on
  Get RPY from rotation matrix : MATLAB Function  TreatAsAtomicUnit=on
  "Get RPY from rotation matrix " : MATLAB Function  TreatAsAtomicUnit=on
  MATLAB Function1 : MATLAB Function  TreatAsAtomicUnit=on
  MATLAB Function2 : MATLAB Function  TreatAsAtomicUnit=on
  MATLAB Function3 : MATLAB Function  TreatAsAtomicUnit=on
  Selector : Selector  NumberOfDimensions=2  InputPortWidth=3  IndexOptions=Index vector (dialog),Index vector (dialog)  Indices=[1:3],4  OutputSizes=1,1
  Selector2 : Selector  NumberOfDimensions=2  InputPortWidth=3  IndexOptions=Index vector (dialog),Index vector (dialog)  Indices=[1:3],[1:3]  OutputSizes=1,1
  Sum : Sum  Inputs=+-|
  wires:
  Demux3/1 -> Base position/1  "b_x"
  Demux3/3 -> Base position/3  "b_z"
  Demux3/2 -> Base position/2  "b_y"
  Selector/1 -> Demux3/1
  w_H_b/1 -> Selector/1
  Demux1/1 -> Base linear velocity/1  "v_x"
  Demux1/3 -> Base linear velocity/3  "v_z"
  Demux2/3 -> Base angular velocity/3  "w_z"
  Demux/2 -> Gain1/1
  Demux2/1 -> Base angular velocity/1  "w_x"
  Demux/1 -> Demux1/1
  Demux2/2 -> Base angular velocity/2  "w_y"
  Gain1/1 -> Demux2/1
  Demux1/2 -> Base linear velocity/2  "v_y"
  "Get RPY from rotation matrix "/1(rollPitchYaw) -> Gain2/1
  Demux5/1 -> Combine Rotations/4(roll_des), Base rotation desired/1  "roll"
  Gain2/1 -> MATLAB Function1/1(rollPitchYaw), Sum/2
  Demux5/2 -> Combine Rotations/5(pitch_des), Base rotation desired/2  "pitch"
  Selector2/1 -> "Get RPY from rotation matrix "/1(w_R_b)
  Demux5/3 -> Combine Rotations/6(yaw_des), Base rotation desired/3  "yaw"
  Demux6/2 -> Base rotation error/2  "pitch"
  Demux6/1 -> Base rotation error/1  "roll"
  Demux6/3 -> Base rotation error/3  "yaw"
  Sum/1 -> MATLAB Function3/1(rollPitchYaw)
  baseTwist/1 -> Demux/1
  rot_vel_acc_jerk_base_des/1 -> Selector2/1
  Gain3/1 -> MATLAB Function2/1(rollPitchYaw), Sum/1
  Demux7/2 -> Combine Rotations/2(pitch), Base rotation/2  "pitch"
  Get RPY from rotation matrix/1(rollPitchYaw) -> Gain3/1
  Demux7/1 -> Combine Rotations/1(roll), Base rotation/1  "roll"
  Demux7/3 -> Combine Rotations/3(yaw), Base rotation/3  "yaw"
  w_R_b/1 -> Get RPY from rotation matrix/1(w_R_b)
  Get RPY error norm/1(rotErr_norm) -> Base rotation error norm/1
  MATLAB Function3/1(RPY_Corr) -> Demux6/1, Get RPY error norm/1(rot_err)
  MATLAB Function1/1(RPY_Corr) -> Demux5/1
  MATLAB Function2/1(RPY_Corr) -> Demux7/1

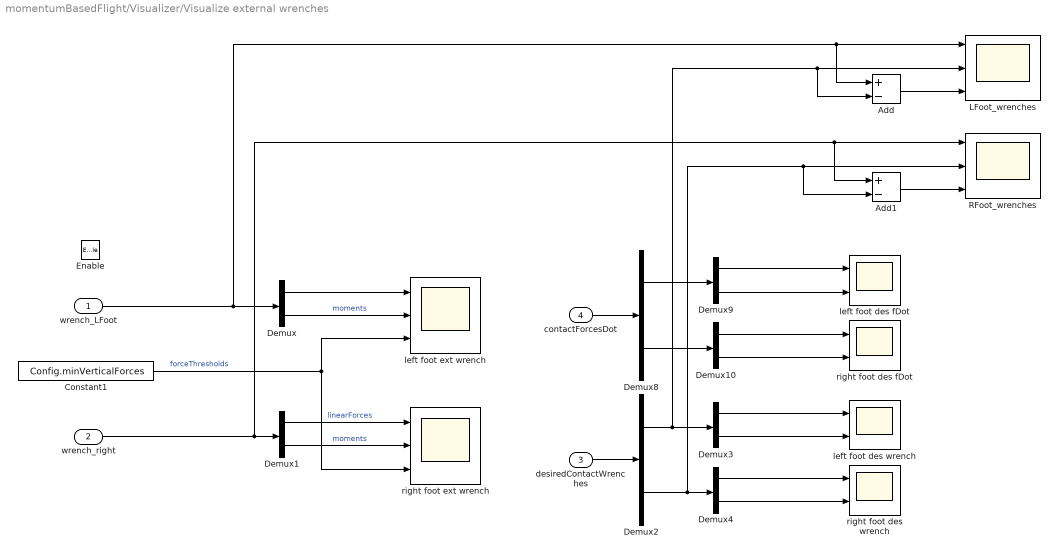
== system momentumBasedFlight/Visualizer/Visualize external wrenches   ==
  wrench_LFoot : Inport
  wrench_right : Inport  Port=2
  desiredContactWrenches : Inport  Port=3
  contactForcesDot : Inport  Port=4
  Enable : EnablePort
  Add : Sum  Inputs=+-
  Add1 : Sum  Inputs=+-
  Constant1 : Constant  Value=Config.minVerticalForces
  Demux{,1,3..4,9..10} (6 alike) : Demux  Outputs=[3;3]
  Demux2 : Demux  Outputs=[6;6]
  Demux8 : Demux  Outputs=[6;6]
  LFoot_wrenches : Scope  NumInputPorts=3
  RFoot_wrenches : Scope  NumInputPorts=3
  left foot des fDot : Scope  NumInputPorts=2
  left foot des wrench : Scope  NumInputPorts=2
  left foot ext wrench : Scope  NumInputPorts=3
  right foot des fDot : Scope  NumInputPorts=2
  right foot des wrench : Scope  NumInputPorts=2
  right foot ext wrench : Scope  NumInputPorts=3
  wires:
  Demux/1 -> left foot ext wrench/1
  Demux/2 -> left foot ext wrench/2  "moments"
  Demux1/1 -> right foot ext wrench/1  "linearForces"
  Demux1/2 -> right foot ext wrench/2  "moments"
  wrench_LFoot/1 -> Add/1, LFoot_wrenches/1, Demux/1
  wrench_right/1 -> Add1/1, RFoot_wrenches/1, Demux1/1
  desiredContactWrenches/1 -> Demux2/1
  Demux2/1 -> Add/2, LFoot_wrenches/2, Demux3/1
  Demux2/2 -> Add1/2, RFoot_wrenches/2, Demux4/1
  Demux4/2 -> right foot des wrench/2
  Demux3/1 -> left foot des wrench/1
  Demux3/2 -> left foot des wrench/2
  Demux8/2 -> Demux10/1
  contactForcesDot/1 -> Demux8/1
  Demux10/2 -> right foot des fDot/2
  Demux8/1 -> Demux9/1
  Demux10/1 -> right foot des fDot/1
  Demux9/2 -> left foot des fDot/2
  Demux9/1 -> left foot des fDot/1
  Constant1/1 -> right foot ext wrench/3, left foot ext wrench/3  "forceThresholds"
  Add/1 -> LFoot_wrenches/3
  Add1/1 -> RFoot_wrenches/3
  Demux4/1 -> right foot des wrench/1

== system momentumBasedFlight/synchronizer/GAZEBO_SYNCHRONIZER ==
  Enable : EnablePort
  Simulator Synchronizer : WBToolboxLibrary/Utilities/Simulator Synchronizer  period=Config.tStep  serverPortName='/clock/rpc'  clientPortName='/WBT_synchronizer/rpc:o'
      settings: SourceProductName=WholeBodyToolbox

== system momentumBasedFlight/synchronizer/REAL_TIME_SYNC ==
  Enable : EnablePort
  Real Time Synchronizer : WBToolboxLibrary/Utilities/Real Time Synchronizer  period=Config.tStep
      settings: SourceProductName=WholeBodyToolbox

== system momentumBasedFlight/FLIGHT CONTROLLER (CORE) V3.0/Dynamics and Kinematics/Dynamic Quantities ==
  posCoM : Inport
  w_H_b : Inport  Port=2
  jointPos : Inport  Port=3
  w_baseTwist : Inport  Port=4
  jointVel : Inport  Port=5
  Compute Centroidal Inertia : Subsystem
  GetBiasForces : WBToolboxLibrary/Model/Dynamics/GetBiasForces
      settings: SourceProductName=WholeBodyToolbox
  MassMatrix : WBToolboxLibrary/Model/Dynamics/MassMatrix
      settings: SourceProductName=WholeBodyToolbox
  Momentum and CentroidalMomentum Matrix : Subsystem
  M : Outport  VectorParamsAs1DForOutWhenUnconnected=off
  "h " : Outport  Port=2  VectorParamsAs1DForOutWhenUnconnected=off
  L : Outport  Port=3  VectorParamsAs1DForOutWhenUnconnected=off
  CMM : Outport  Port=4  VectorParamsAs1DForOutWhenUnconnected=off
  w_I_c : Outport  Port=5  VectorParamsAs1DForOutWhenUnconnected=off
  tag scope: momentum=global
  wires:
  posCoM/1 -> Compute Centroidal Inertia/3(posCoM)  "com_pos"
  Compute Centroidal Inertia/1(w_I_c) -> w_I_c/1
  jointPos/1 -> Momentum and CentroidalMomentum Matrix/2(jointPos), MassMatrix/2, GetBiasForces/2
  Momentum and CentroidalMomentum Matrix/1(L) -> [momentum], L/1
  Momentum and CentroidalMomentum Matrix/2(CMM) -> CMM/1
  GetBiasForces/1 -> "h "/1
  MassMatrix/1 -> M/1, Compute Centroidal Inertia/1(M)
  jointVel/1 -> GetBiasForces/4, Momentum and CentroidalMomentum Matrix/4(jointVel)
  w_baseTwist/1 -> GetBiasForces/3, Momentum and CentroidalMomentum Matrix/3(w_baseTwist)
  w_H_b/1 -> MassMatrix/1, Compute Centroidal Inertia/2(w_H_b), GetBiasForces/1, Momentum and CentroidalMomentum Matrix/1(w_H_b)  "w_H_b"
